simulink model "Experiment - 6_Labwork"  (R2016a)
settings: Solver=VariableStepAuto  StartTime=0.0  StopTime=10  RelTol=1e-3
settings Model: Creator=AIUB  LastModifiedBy=AIUB

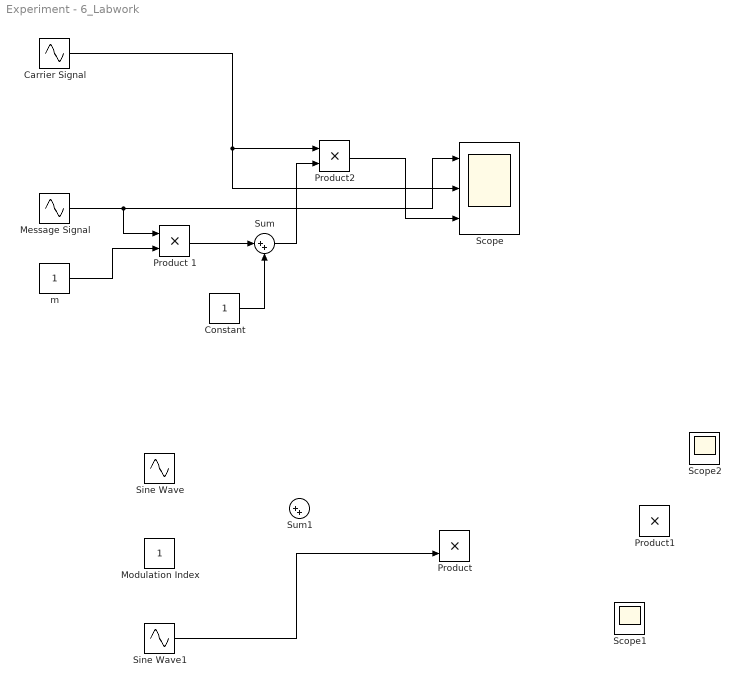
== system Experiment - 6_Labwork ==
  Carrier Signal : Sin  Frequency=100  SampleTime=0
  Constant : Constant
  Message Signal : Sin  Frequency=10  SampleTime=0
  Modulation Index : Constant
  Product : Product
  Product 1 : Product
  Product1 : Product
  Product2 : Product
  Scope : Scope  NumInputPorts=3
  Scope1 : Scope
  Scope2 : Scope
  Sine Wave : Sin  SampleTime=0
  Sine Wave1 : Sin  SampleTime=0
  Sum : Sum  Inputs=|++
  Sum1 : Sum  Inputs=|++
  m : Constant
  wires:
  m/1 -> Product 1/2
  Product 1/1 -> Sum/1
  Constant/1 -> Sum/2
  Carrier Signal/1 -> Scope/2, Product2/1
  Sum/1 -> Product2/2
  Sine Wave1/1 -> Product/2
  Product2/1 -> Scope/3
  Message Signal/1 -> Scope/1, Product 1/1
